simulink library "rayTrace_ul"  (R2018b)
settings: Solver=VariableStepAuto  StartTime=0.0  StopTime=10.0  RelTol=1e-3
values from neighbouring files (symbols this model uses):
  grnd2CamRotMat = calculateRotationMatrix(     camEulAngles_rad(1),camEulAngles_rad(2),camEulAngles_rad(3))    [rayTrace_init.m]
settings Model: Creator=MAE-NCSUCORE  LastModifiedBy=mcobb

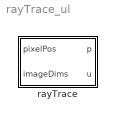
== system rayTrace_ul ==
  rayTrace : Subsystem  mask{camPosVec_cm=[5 0 0], camEulAngles_deg=[0 90 0], dist2Glass_cm=1, indOfRefVec=[1 1 1], glassNormalVec=[1 0 0], glassThickness_cm=0.1, camFOV_deg=[20 20]}
      mask prompts: camPosVec_cm "Camera Position Vector, cm"; camEulAngles_deg "Camera Euler Angles, deg"; dist2Glass_cm "Distance to glass, cm"; indOfRefVec "Indices of refraction [air glass water]"; glassNormalVec "Glass outwards normal unit vec"; glassThickness_cm "Glass thickness, cm"; camFOV_deg "Camera field of view angles,deg  [horiz vert]"
      mask init:
      | rayTrace_init

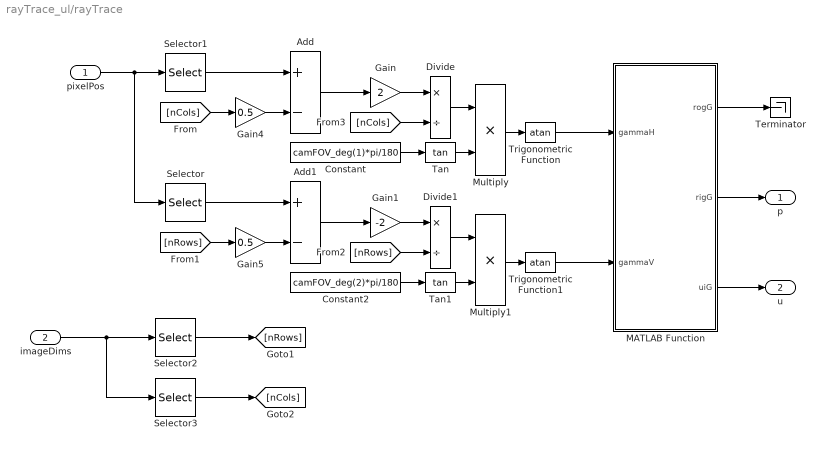
== system rayTrace_ul/rayTrace ==
  pixelPos : Inport
  imageDims : Inport  Port=2
  Add : Sum  Inputs=+-
  Add1 : Sum  Inputs=+-
  Constant : Constant  Value=camFOV_deg(1)*pi/180
  Constant2 : Constant  Value=camFOV_deg(2)*pi/180
  Divide : Product  Inputs=*/
  Divide1 : Product  Inputs=*/
  Gain : Gain  Gain=2
  Gain1 : Gain  Gain=-2
  Gain4 : Gain  Gain=0.5
  Gain5 : Gain  Gain=0.5
  MATLAB Function : MATLAB Function  TreatAsAtomicUnit=on
  Multiply : Product
  Multiply1 : Product
  Selector : Selector  InputPortWidth=2  IndexOptions=Index vector (dialog)  Indices=1  OutputSizes=1
  Selector1 : Selector  InputPortWidth=2  IndexOptions=Index vector (dialog)  Indices=2  OutputSizes=1
  Selector2 : Selector  InputPortWidth=2  IndexOptions=Index vector (dialog)  Indices=1  OutputSizes=1
  Selector3 : Selector  InputPortWidth=2  IndexOptions=Index vector (dialog)  Indices=2  OutputSizes=1
  Tan : Trigonometry  Operator=tan
  Tan1 : Trigonometry  Operator=tan
  Terminator : Terminator
  Trigonometric Function : Trigonometry  Operator=atan
  Trigonometric Function1 : Trigonometry  Operator=atan
  p : Outport
  u : Outport  Port=2
  wires:
  MATLAB Function/2(rigG) -> p/1
  MATLAB Function/3(uiG) -> u/1
  MATLAB Function/1(rogG) -> Terminator/1
  Trigonometric Function/1 -> MATLAB Function/1(gammaH)
  Multiply/1 -> Trigonometric Function/1
  Tan/1 -> Multiply/2
  Constant/1 -> Tan/1
  Divide/1 -> Multiply/1
  Gain/1 -> Divide/1
  [nCols] -> Divide/2
  Gain1/1 -> Divide1/1
  [nRows] -> Divide1/2
  Constant2/1 -> Tan1/1
  Trigonometric Function1/1 -> MATLAB Function/2(gammaV)
  Multiply1/1 -> Trigonometric Function1/1
  Tan1/1 -> Multiply1/2
  Divide1/1 -> Multiply1/1
  Add/1 -> Gain/1
  [nCols] -> Gain4/1
  Gain4/1 -> Add/2
  [nRows] -> Gain5/1
  Selector/1 -> Add1/1
  Gain5/1 -> Add1/2
  Add1/1 -> Gain1/1
  pixelPos/1 -> Selector/1, Selector1/1
  Selector1/1 -> Add/1
  Selector3/1 -> [nCols]
  Selector2/1 -> [nRows]
  imageDims/1 -> Selector3/1, Selector2/1

== matlab function rayTrace_ul/rayTrace/MATLAB Function ==
  data: rogG output; rigG output; gammaH input; gammaV input; uiG output; camPosVec_cm parameter; grnd2CamRotMat parameter; dist2Glass_cm parameter; indOfRefVec parameter; glassNormalVec parameter; glassThickness_cm parameter
function [rogG,rigG,uiG] = ...
    rayTrace(gammaH,gammaV,camPosVec_cm,grnd2CamRotMat,dist2Glass_cm,...
    indOfRefVec,glassNormalVec,glassThickness_cm)

[rogG,rigG,uiG] = ...
    rayTrace(camPosVec_cm,grnd2CamRotMat,dist2Glass_cm,gammaH,gammaV,...
    indOfRefVec,glassNormalVec,glassThickness_cm);
